simulink model "PMT_AI_Env_Version1_MatlabRL"  (R2025a)
settings: Solver=ode4  StartTime=0.0  StopTime=10  FixedStep=0.00001  RelTol=1e-3
libraries: instrumentlib x2, slpidlib x1
settings Model: Creator=30623  LastModifiedBy=Administrator

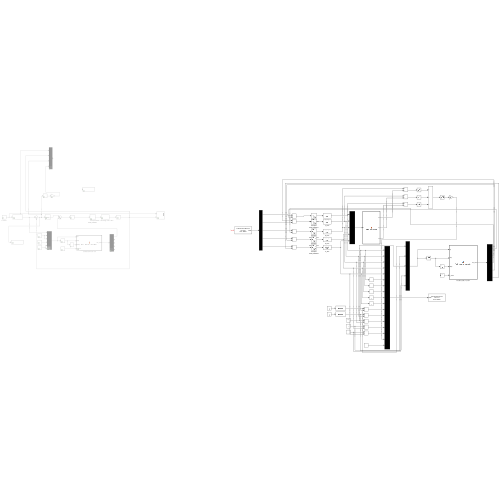
[thumbnail: Simulink's stored preview of the top-level diagram]
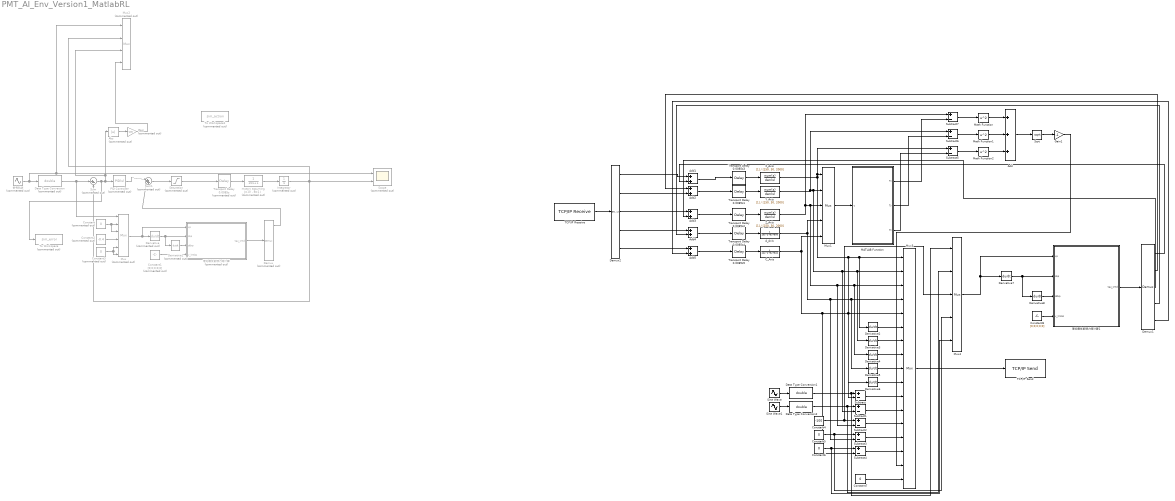
== system PMT_AI_Env_Version1_MatlabRL ==
  A_Axis : TransferFcn  Denominator=[20, 5, 500]
  Abs : Abs  Commented=on  SaturateOnIntegerOverflow=off
  Add : Sum  Inputs=+++
  Add{1..5} (5 alike) : Sum
  C_Axis : TransferFcn  Denominator=[20, 5, 500]
  Constant : Constant  Commented=on  Value=0
  Constant1 : Constant  Commented=on  Value=[0;0;0;0;0]
  Constant2 : Constant  Commented=on  Value=-0.4
  Constant3 : Constant  Commented=on  Value=0
  Constant4 : Constant  Value=-100
  Constant5 : Constant  Value=0
  Constant6 : Constant  Value=0
  Constant7 : Constant  Value=0
  Constant8 : Constant  Value=[0;0;0;0;0]
  Data Type Conversion : DataTypeConversion  Commented=on  OutDataTypeStr=double  SaturateOnIntegerOverflow=off  RndMeth=Floor
  Data Type Conversion1 : DataTypeConversion  OutDataTypeStr=double  SaturateOnIntegerOverflow=off  RndMeth=Floor
  Data Type Conversion2 : DataTypeConversion  OutDataTypeStr=double  SaturateOnIntegerOverflow=off  RndMeth=Floor
  Demux : Demux  Commented=on  Outputs=5
  Demux1 : Demux  Outputs=5
  Demux2 : Demux  Outputs=5
  Derivative : Derivative  Commented=on
  Derivative1 : Derivative  Commented=on
  Derivative{2..8} (7 alike) : Derivative
  Gain : Gain  Commented=on  Gain=-100
  Gain1 : Gain  Gain=-1
  Integrator : Integrator  Commented=on
  MATLAB Function : MATLAB Function  TreatAsAtomicUnit=on
  Math Function : Math  Operator=square
  Math Function1 : Math  Operator=square
  Math Function2 : Math  Operator=square
  Mux : Mux  Commented=on  Inputs=6
  Mux1 : Mux  Inputs=5
  Mux2 : Mux  Commented=on
  Mux3 : Mux  Inputs=17
  Mux4 : Mux  Inputs=5
  PID Controller : slpidlib/PID Controller  Commented=on  Controller=PID  Form=Parallel  TimeDomain=Continuous-time  UseExternalTs=off  SampleTime=-1  IntegratorMethod=Forward Euler  FilterMethod=Forward Euler  ControllerParametersSource=internal  P=1  I=1  UseKiTs=off  D=0  UseExternalDerivativeSource=off  N=100  UseFilter=on  TunerSelectOption=Transfer Function Based (PID Tuner App)  InitialConditionSource=internal  InitialConditionForIntegrator=0  InitialConditionForFilter=0  DifferentiatorICPrevScaledInput=0  ExternalReset=none  TrackingMode=off  Kt=1  LimitOutput=off  SatLimitsSource=internal  UpperSaturationLimit=inf  LowerSaturationLimit=-inf  LinearizeAsGain=on  AntiWindupMode=none  Kb=1  LimitIntegrator=off  UpperIntegratorSaturationLimit=inf  LowerIntegratorSaturationLimit=-inf  POutMin=[]  POutMax=[]  IOutMin=[]  IOutMax=[]  DOutMin=[]  DOutMax=[]  NOutMin=[]  NOutMax=[]  SumOutMin=[]  SumOutMax=[]  SaturationOutMin=[]  SaturationOutMax=[]  PParamMin=[]  PParamMax=[]  IParamMin=[]  IParamMax=[]  DParamMin=[]  DParamMax=[]  NParamMin=[]  NParamMax=[]  KbParamMin=[]  KbParamMax=[]  KtParamMin=[]  KtParamMax=[]  KbOutMin=[]  KbOutMax=[]  KtOutMin=[]  KtOutMax=[]  IntegratorOutMin=[]  IntegratorOutMax=[]  FilterOutMin=[]  FilterOutMax=[]  SumI1OutMin=[]  SumI1OutMax=[]  SumI2OutMin=[]  SumI2OutMax=[]  SumI3OutMin=[]  SumI3OutMax=[]  SumI4OutMin=[]  SumI4OutMax=[]  SumDOutMin=[]  SumDOutMax=[]  DifferentiatorOutMin=[]  DifferentiatorOutMax=[]  FilterDiffOutCoefMin=[]  FilterDiffOutCoefMax=[]  ReciprocalOutMin=[]  ReciprocalOutMax=[]  SumDenOutMin=[]  SumDenOutMax=[]  SumNumOutMin=[]  SumNumOutMax=[]  DivideOutMin=[]  DivideOutMax=[]  UdiffTsProdOutMin=[]  UdiffTsProdOutMax=[]  NTsProdOutMin=[]  NTsProdOutMax=[]  UintegralTsProdOutMin=[]  UintegralTsProdOutMax=[]  UngainTsProdOutMin=[]  UngainTsProdOutMax=[]  ClampingZeroOutDataTypeStr=Inherit: Inherit via back propagation  ClampingZeroOutMin=[]  ClampingZeroOutMax=[]  FilterDenConstantOutDataTypeStr=Inherit: Inherit via back propagation  FilterDenConstantOutMin=[]  FilterDenConstantOutMax=[]  PCopyOutDataTypeStr=Inherit: Inherit via back propagation  PCopyOutMin=[]  PCopyOutMax=[]  NCopyOutDataTypeStr=Inherit: Inherit via back propagation  NCopyOutMin=[]  NCopyOutMax=[]  IntegratorContinuousStateAttributes=''  IntegratorStateMustResolveToSignalObject=off  IntegratorRTWStateStorageClass=Auto  FilterContinuousStateAttributes=''  FilterStateMustResolveToSignalObject=off  FilterRTWStateStorageClass=Auto  ParallelPVariant=InternalParameters  IdealPVariant=Disabled  IVariant=InternalParameters  DVariant=InternalParameters  IntegratorVariant=Continuous  SatVariant=Disabled  AWVariant=Passthrough  PCopyVariant=Disabled  TRVariant=Disabled  FdbkBlocksVariant=Forward  IdealPFdbkVariant=Disabled  SatFdbkVariant=Disabled  DerivativeFilterVariant=ContFilter  NVariant=InternalParameters  NCopyVariant=Disabled  FilterICVariant=InternalICsFilter  IntegratorICVariant=InternalICs  ExternalResetVariant=Disabled  TRSumVariant=Passthrough  SumFdbkVariant=Disabled  SumVariant=Sum_PID  TsampFilterVariant=InternalTs  TsampNgainVariant=Passthrough  TsampIntegralVariant=Disabled_SignalSpec  ExternalSaturationOutDataTypeStr=Inherit: Same as second input  DerivativeSourceVariant=ErrorSignal  PreIntVariant=InternalPreInt
  Saturation : Saturate  Commented=on  UpperLimit=500  LowerLimit=-500
  Scope : Scope  Commented=on  NumInputPorts=2
      settings: ActiveDisplayYMinimum=-50413.733349400849  ActiveDisplayYMaximum=34151.372945794108
  Sine Wave : Sin  SampleTime=0
  Sine Wave1 : Sin  SampleTime=0
  Sqrt : Sqrt
  Subtract{,1..7} (8 alike) : Sum  Inputs=+-
  Sum : Sum  Commented=on  Inputs=|+-
  Sum1 : Sum  Commented=on  Inputs=|+++
  TCP/IP Receive : instrumentlib/TCP//IP Receive  Host=127.0.0.1  Port=50001  DataSize=5  DataType=double  ASCIIFormatting=%f  Terminator=LF  CustomTerminator=10  ByteOrder=big-endian  EnableBlockingMode=on  Timeout=30  SampleTime=0.01  SimulateUsing=Interpreted execution
  TCP/IP Send : instrumentlib/TCP//IP Send  Host=127.0.0.1  Port=50000  ByteOrder=big-endian  EnableBlockingMode=on  Timeout=10  TransferDelay=on  SimulateUsing=Interpreted execution
  To Workspace : ToWorkspace  Commented=on  VariableName=sim_error  SaveFormat=Timeseries  SampleTime=-1
  To Workspace1 : ToWorkspace  Commented=on  VariableName=sim_action  SaveFormat=Timeseries  SampleTime=-1
  Transport Delay 0.0085s : TransportDelay  Commented=on  DelayTime=0.00875
  Transport Delay 0.0085s{1..5} (5 alike) : TransportDelay  DelayTime=0.00875
  X_Axis : TransferFcn  Denominator=[150, 30, 2000]
  Y_Axis : TransferFcn  Denominator=[150, 30, 2000]
  Z_Axis : TransferFcn  Denominator=[150, 30, 2000]
  motor（assuming J=10，B=1） : TransferFcn  Commented=on  Denominator=[10 1]
  参考轨迹 : Sin  Commented=on  Amplitude=0.05  Frequency=2  SampleTime=0
  理论最优前馈力矩计算 : MATLAB Function  Commented=on  TreatAsAtomicUnit=on
  理论最优前馈力矩计算1 : MATLAB Function  TreatAsAtomicUnit=on
  wires:
  Transport Delay 0.0085s/1 -> motor（assuming J=10，B=1）/1
  Data Type Conversion/1 -> Mux/1, Sum/1
  Sum/1 -> To Workspace/1, Abs/1, Mux2/3, PID Controller/1
  motor（assuming J=10，B=1）/1 -> Integrator/1
  Integrator/1 -> Mux2/2, Sum/2, Scope/2
  PID Controller/1 -> Sum1/1
  Constant/1 -> Mux/3, Mux/2
  Mux/1 -> 理论最优前馈力矩计算/1(xp), Derivative/1
  Derivative/1 -> Derivative1/1, 理论最优前馈力矩计算/2(dxp)
  Derivative1/1 -> 理论最优前馈力矩计算/3(ddxp)
  Constant1/1 -> 理论最优前馈力矩计算/4(v_limbs)
  理论最优前馈力矩计算/1(tau_cmd) -> Demux/1
  Demux/1 -> Sum1/2
  参考轨迹/1 -> Mux2/1, Scope/1, Data Type Conversion/1
  Constant2/1 -> Mux/4
  Constant3/1 -> Mux/6, Mux/5
  Sum1/1 -> Saturation/1
  Saturation/1 -> Transport Delay 0.0085s/1
  Abs/1 -> Gain/1
  Gain/1 -> Mux2/4
  Z_Axis/1 -> Subtract7/1, Subtract2/2, Derivative4/1, Mux3/3, Mux1/3
  A_Axis/1 -> Mux1/4, Subtract3/2, Derivative5/1, Mux3/4
  C_Axis/1 -> Mux1/5, Subtract4/2, Derivative6/1, Mux3/5
  Mux1/1 -> MATLAB Function/1(u)
  X_Axis/1 -> Subtract5/1, Mux1/1, Subtract/2, Derivative2/1, Mux3/1
  Y_Axis/1 -> Mux1/2, Subtract1/2, Derivative3/1, Mux3/2, Subtract6/1
  Transport Delay 0.0085s3/1 -> X_Axis/1
  Transport Delay 0.0085s1/1 -> Y_Axis/1
  Transport Delay 0.0085s2/1 -> Z_Axis/1
  Transport Delay 0.0085s4/1 -> A_Axis/1
  Transport Delay 0.0085s5/1 -> C_Axis/1
  Derivative2/1 -> Mux3/6
  Derivative3/1 -> Mux3/7
  Derivative4/1 -> Mux3/8
  Derivative5/1 -> Mux3/9
  Derivative6/1 -> Mux3/10
  Sine Wave/1 -> Data Type Conversion1/1
  Constant4/1 -> Mux4/3, Subtract2/1
  Constant5/1 -> Mux4/4, Subtract3/1
  Constant6/1 -> Mux4/5, Subtract4/1
  Subtract/1 -> Mux3/11
  Subtract1/1 -> Mux3/12
  Subtract2/1 -> Mux3/13
  Subtract3/1 -> Mux3/14
  Subtract4/1 -> Mux3/15
  MATLAB Function/1(Tx) -> Subtract7/2
  MATLAB Function/2(Ty) -> Subtract6/2
  MATLAB Function/3(Tz) -> Subtract5/2
  Subtract7/1 -> Math Function/1
  Subtract6/1 -> Math Function1/1
  Subtract5/1 -> Math Function2/1
  Math Function/1 -> Add/1
  Math Function1/1 -> Add/2
  Math Function2/1 -> Add/3
  Add/1 -> Sqrt/1
  Sqrt/1 -> Gain1/1
  Gain1/1 -> Mux3/16
  Constant7/1 -> Mux3/17
  Mux3/1 -> TCP/IP Send/1
  Mux4/1 -> 理论最优前馈力矩计算1/1(xp), Derivative7/1
  Derivative7/1 -> Derivative8/1, 理论最优前馈力矩计算1/2(dxp)
  Derivative8/1 -> 理论最优前馈力矩计算1/3(ddxp)
  Constant8/1 -> 理论最优前馈力矩计算1/4(v_limbs)
  理论最优前馈力矩计算1/1(tau_cmd) -> Demux1/1
  Demux1/1 -> Add1/2
  Add1/1 -> Transport Delay 0.0085s3/1
  Demux1/2 -> Add2/1
  Add2/1 -> Transport Delay 0.0085s1/1
  Add3/1 -> Transport Delay 0.0085s2/1
  Add4/1 -> Transport Delay 0.0085s4/1
  Add5/1 -> Transport Delay 0.0085s5/1
  Demux1/3 -> Add3/2
  Demux1/4 -> Add4/2
  Demux1/5 -> Add5/2
  Data Type Conversion1/1 -> Mux4/1, Subtract/1
  Data Type Conversion2/1 -> Mux4/2, Subtract1/1
  Sine Wave1/1 -> Data Type Conversion2/1
  ? -> ?
  TCP/IP Receive/1 -> Demux2/1
  Demux2/1 -> Add1/1
  Demux2/2 -> Add2/2
  Demux2/3 -> Add3/1
  Demux2/4 -> Add4/1
  Demux2/5 -> Add5/1

== matlab function PMT_AI_Env_Version1_MatlabRL/MATLAB Function ==
  data: u input; Tx output; Ty output; Tz output
function [Tx, Ty, Tz] = FiveAxisKinematics(u)
    % 解析输入的 5 个实际物理量
    x = u(1); y = u(2); z = u(3); 
    a = u(4); c = u(5);
    
    % --- D-H 齐次变换矩阵推导 (基于 AC 摇篮台机床) ---
    % 1. 直线平移矩阵
    Trans = [1 0 0 x;
             0 1 0 y;
             0 0 1 z;
             0 0 0 1];
             
    % 2. A 轴旋转矩阵 (绕 X 轴)
    RotA = [1       0        0 0;
            0  cos(a)  -sin(a) 0;
            0  sin(a)   cos(a) 0;
            0       0        0 1];
           
    % 3. C 轴旋转矩阵 (绕 Z 轴)
    RotC = [cos(c) -sin(c) 0 0;
            sin(c)  cos(c) 0 0;
            0       0      1 0;
            0       0      0 1];
           
    % 4. 运动链合成
    T_total = Trans * RotA * RotC; 
    
    % 5. 计算真实的刀尖点 (假设初始刀具长度为100mm，沿Z轴负方向)
    P_tool = T_total * [0; 0; -100; 1];
    
    % 输出三维空间中真实的刀尖点坐标
    Tx = P_tool(1);
    Ty = P_tool(2);
    Tz = P_tool(3);
end

== matlab function PMT_AI_Env_Version1_MatlabRL/理论最优前馈力矩计算 ==
  data: xp input; tau_cmd output; dxp input; ddxp input; v_limbs input
%理论最优前馈力矩计算
function tau_cmd = PMT_Dynamics_Controller(xp, dxp, ddxp, v_limbs)
    % 输入: 
    % xp: [x, y, z, phi, theta]' 动平台位姿 (T&T angles)
    % dxp: [v_x, v_y, v_z, w_x, w_y, w_z]' 动平台速度 
    % ddxp: [a_x, a_y, a_z, dw_x, dw_y, dw_z]' 动平台加速度 
    % v_limbs: [v1, v2, v3, v4, v5]' 五个驱动支链的实际线速度 (用于计算摩擦力) 
    % 输出:
    % tau_cmd: [tau1, tau2, tau3, tau4, tau5]' 五个伺服电机的目标前馈力矩
    % 定义反对称矩阵算子 S(v)，用于计算叉乘 
    S = @(v) [0, -v(3), v(2); v(3), 0, -v(1); -v(2), v(1), 0];
    
    %% 1. 物理与几何参数化
    % 动平台真实辨识惯性参数 (摘自解老师论文 Table 2) 
    m_p = 45.32; 
    mp_es = 8.384; 
    I_xx = 6.24e-4; I_yy = 6.24e-4; I_zz = 1.03e-4;
    I_p_matrix = diag([I_xx, I_yy, I_zz]); % 忽略极小的耦合项 
    g_vec = [0; 0; -9.81]; 
    
    % 驱动支链真实辨识摩擦力参数 (摘自论文 Table 1: [Tc, Ts, vs, Bv]) 
    Fric_Params = [
        186.21, 291.52, -1.87, 3.027; % Limb 1
        244.34, 372.97,  1.26, 3.766; % Limb 2
        187.89, 273.38,  1.35, 3.006; % Limb 3
        226.99, 314.07,  1.30, 3.489; % Limb 4
        224.82, 312.41,  2.69, 2.696  % Limb 5
    ];
    
    % 虚拟几何参数 (因原论文未公开，用于 DRL 环境预研构建)
    R_b = 0.5; % 基座分布半径 0.5m
    b = [
        0,  R_b*cos(pi/4), R_b*cos(3*pi/4), R_b*cos(5*pi/4), R_b*cos(7*pi/4);
        0,  R_b*sin(pi/4), R_b*sin(3*pi/4), R_b*sin(5*pi/4), R_b*sin(7*pi/4);
        0,  0,             0,               0,               0
    ];
    
    R_p = 0.15; % 动平台铰链分布半径 0.15m
    H_tool = -0.1; % 刀尖到平台铰链面的 Z 向距离
    p_local = [
        0,       R_p*cos(pi/4), R_p*cos(3*pi/4), R_p*cos(5*pi/4), R_p*cos(7*pi/4);
        0,       R_p*sin(pi/4), R_p*sin(3*pi/4), R_p*sin(5*pi/4), R_p*sin(7*pi/4);
        H_tool,  H_tool,        H_tool,          H_tool,          H_tool
    ];
    
    %% 2. 运动学正解与雅可比矩阵构建 
    % (1) 计算旋转矩阵 R (基于 T&T angles, Eq. A-1) 
    phi = xp(4); theta = xp(5);
    p_vec = [cos(phi)*sin(theta); sin(phi)*sin(theta); cos(theta)];
    
    % 依据原论文的投影法生成正交旋转矩阵 R 
    O_B1 = b(:,1); 
    n_vec = cross(O_B1, p_vec); 
    if norm(n_vec) < 1e-6
        n_vec = [1;0;0]; % 奇异保护
    else
        n_vec = n_vec / norm(n_vec);
    end
    o_vec = cross(p_vec, n_vec);
    R = [n_vec, o_vec, p_vec];
    
    % (2) 运动传递雅可比 J_t (5x6 矩阵) 
    J_t = zeros(5, 6); 
    l_unit_all = zeros(3, 5); % 保存单位方向向量备用
    L_all = zeros(1, 5);      % 保存支链长度备用
    p_global_all = zeros(3, 5); % 保存全局坐标备用
    for i = 1:5
        p_i_global = R * p_local(:, i); % Eq. A-2 
        p_global_all(:, i) = p_i_global;
        
        l_vec = (xp(1:3) + p_i_global) - b(:, i); % Eq. A-3 
        L_i = norm(l_vec);
        L_all(i) = L_i;
        l_unit = l_vec / L_i; % Eq. A-3 
        l_unit_all(:, i) = l_unit;
        
        J_t(i, :) = [l_unit', (cross(p_i_global, l_unit))']; % 组装 J_t 
    end
    
    % (3) 约束雅可比 J_c (1x6 矩阵，第一条 SPR 支链提供的一维约束) 
    J_c = [n_vec', (L_all(1) * cross(n_vec, l_unit_all(:,1)) + cross(p_global_all(:,1), n_vec))'];
    % 组装完整满秩雅可比矩阵 J_a (6x6 矩阵) 
    J_a = [J_t; J_c]; 
    
    %% 3. 动力学受力分析 (附录 A.2 解老师用到了虚功原理) 
    % (1) 动平台惯性力和重力 F_p (Eq. A-12) 
    w_p = dxp(4:6);   % 角速度
    dw_p = ddxp(4:6); % 角加速度
    a_c = ddxp(1:3);  % 线加速度
    
    F_p_trans = m_p * g_vec - m_p * a_c; 
    F_p_rot = -I_p_matrix * dw_p - cross(w_p, I_p_matrix * w_p);
    F_p = [F_p_trans; F_p_rot]; % 6x1 向量
    
    % (2) 支链惯性力简化 (为提高仿真速度，此处将支链质量等效附加到平台上)
    F_limbs_total = zeros(6, 1); 
    
    %% 4. 虚功反解理论刚体力矩 
    % 求解: J_a' * [tau_ideal; F_constraint] = - F_p 
   Tau_and_Constraint = pinv(J_a') * (-F_p - F_limbs_total);
    tau_ideal = Tau_and_Constraint(1:5); % 提取前5个主动电机的理论力矩
    
    %% 5. Stribeck 非线性摩擦力补偿 (Eq. 4) 
    f_friction = zeros(5, 1);
    for i = 1:5
        v = v_limbs(i);
        Tc = Fric_Params(i, 1);
        Ts = Fric_Params(i, 2);
        vs = Fric_Params(i, 3);
        Bv = Fric_Params(i, 4);
       
        f_friction(i) = (Tc + (Ts - Tc) * exp(-(v/vs)^2)) * sign(v) + Bv * v; 
    end
    
    %% 6. 输出最终前馈力矩指令 
    tau_cmd = tau_ideal + f_friction;
end

== matlab function PMT_AI_Env_Version1_MatlabRL/理论最优前馈力矩计算1 ==
  data: xp input; tau_cmd output; dxp input; ddxp input; v_limbs input
%理论最优前馈力矩计算
function tau_cmd = PMT_Dynamics_Controller(xp, dxp, ddxp, v_limbs)
    % 输入: 
    % xp: [x, y, z, phi, theta]' 动平台位姿 (T&T angles)
    % dxp: [v_x, v_y, v_z, dphi, dtheta]' 或 [v_x, v_y, v_z, w_x, w_y, w_z]' 动平台速度 
    % ddxp: [a_x, a_y, a_z, ddphi, ddtheta]' 或 [a_x, a_y, a_z, dw_x, dw_y, dw_z]' 动平台加速度 
    % v_limbs: [v1, v2, v3, v4, v5]' 五个驱动支链的实际线速度 (用于计算摩擦力) 
    % 输出:
    % tau_cmd: [tau1, tau2, tau3, tau4, tau5]' 五个伺服电机的目标前馈力矩
    
    % 定义反对称矩阵算子 S(v)，用于计算叉乘 
    S = @(v) [0, -v(3), v(2); v(3), 0, -v(1); -v(2), v(1), 0];
    
    %% 1. 物理与几何参数化
    % 动平台真实辨识惯性参数 (摘自解老师论文 Table 2) 
    m_p = 45.32; 
    mp_es = 8.384; 
    I_xx = 6.24e-4; I_yy = 6.24e-4; I_zz = 1.03e-4;
    I_p_matrix = diag([I_xx, I_yy, I_zz]); % 忽略极小的耦合项 
    g_vec = [0; 0; -9.81]; 
    
    % 驱动支链真实辨识摩擦力参数 (摘自论文 Table 1: [Tc, Ts, vs, Bv]) 
    Fric_Params = [
        186.21, 291.52, -1.87, 3.027; % Limb 1
        244.34, 372.97,  1.26, 3.766; % Limb 2
        187.89, 273.38,  1.35, 3.006; % Limb 3
        226.99, 314.07,  1.30, 3.489; % Limb 4
        224.82, 312.41,  2.69, 2.696  % Limb 5
    ];
    
    % 虚拟几何参数 (因原论文未公开，用于 DRL 环境预研构建)
    R_b = 0.5; % 基座分布半径 0.5m
    b = [
        0,  R_b*cos(pi/4), R_b*cos(3*pi/4), R_b*cos(5*pi/4), R_b*cos(7*pi/4);
        0,  R_b*sin(pi/4), R_b*sin(3*pi/4), R_b*sin(5*pi/4), R_b*sin(7*pi/4);
        0,  0,             0,               0,               0
    ];
    
    R_p = 0.15; % 动平台铰链分布半径 0.15m
    H_tool = -0.1; % 刀尖到平台铰链面的 Z 向距离
    p_local = [
        0,       R_p*cos(pi/4), R_p*cos(3*pi/4), R_p*cos(5*pi/4), R_p*cos(7*pi/4);
        0,       R_p*sin(pi/4), R_p*sin(3*pi/4), R_p*sin(5*pi/4), R_p*sin(7*pi/4);
        H_tool,  H_tool,        H_tool,          H_tool,          H_tool
    ];
    
    %% 2. 运动学正解与雅可比矩阵构建 
    % (1) 计算旋转矩阵 R (基于 T&T angles, Eq. A-1) 
    phi = xp(4); theta = xp(5);
    p_vec = [cos(phi)*sin(theta); sin(phi)*sin(theta); cos(theta)];
    
    % 依据原论文的投影法生成正交旋转矩阵 R 
    O_B1 = b(:,1); 
    n_vec = cross(O_B1, p_vec); 
    if norm(n_vec) < 1e-6
        n_vec = [1;0;0]; % 奇异保护
    else
        n_vec = n_vec / norm(n_vec);
    end
    o_vec = cross(p_vec, n_vec);
    R = [n_vec, o_vec, p_vec];
    
    % (2) 运动传递雅可比 J_t (5x6 矩阵) 
    J_t = zeros(5, 6); 
    l_unit_all = zeros(3, 5); % 保存单位方向向量备用
    L_all = zeros(1, 5);      % 保存支链长度备用
    p_global_all = zeros(3, 5); % 保存全局坐标备用
    for i = 1:5
        p_i_global = R * p_local(:, i); % Eq. A-2 
        p_global_all(:, i) = p_i_global;
        
        l_vec = (xp(1:3) + p_i_global) - b(:, i); % Eq. A-3 
        L_i = norm(l_vec);
        L_all(i) = L_i;
        l_unit = l_vec / L_i; % Eq. A-3 
        l_unit_all(:, i) = l_unit;
        
        J_t(i, :) = [l_unit', (cross(p_i_global, l_unit))']; % 组装 J_t 
    end
    
    % (3) 约束雅可比 J_c (1x6 矩阵，第一条 SPR 支链提供的一维约束) 
    J_c = [n_vec', (L_all(1) * cross(n_vec, l_unit_all(:,1)) + cross(p_global_all(:,1), n_vec))'];
    % 组装完整满秩雅可比矩阵 J_a (6x6 矩阵) 
    J_a = [J_t; J_c]; 
    
    %% 3. 动力学受力分析 
    % ----- 【修复区域：自适应维度转换】 -----
    % 判断速度输入维度
    if length(dxp) == 5
        % 如果输入是 5 维：[vx, vy, vz, dphi, dtheta]
        dphi = dxp(4); 
        dtheta = dxp(5);
        % 映射到 3D 空间角速度
        w_p = [0; 0; dphi] + dtheta * n_vec; 
    else
        % 如果输入已经是 6 维：[vx, vy, vz, wx, wy, wz]
        w_p = dxp(4:6);
    end

    % 判断加速度输入维度
    if length(ddxp) == 5
        a_c = ddxp(1:3);
        ddphi = ddxp(4);
        ddtheta = ddxp(5);
        % 映射到 3D 空间角加速度
        dw_p = [0; 0; ddphi] + ddtheta * n_vec; 
    else
        a_c = ddxp(1:3);
        dw_p = ddxp(4:6);
    end
    % -----------------------------------------

    F_p_trans = m_p * g_vec - m_p * a_c; 
    F_p_rot = -I_p_matrix * dw_p - cross(w_p, I_p_matrix * w_p);
    F_p = [F_p_trans; F_p_rot]; % 此时 F_p 稳定输出为 6x1 向量
    
    % (2) 支链惯性力简化 (为提高仿真速度，此处将支链质量等效附加到平台上)
    F_limbs_total = zeros(6, 1); 
    
    %% 4. 虚功反解理论刚体力矩 
    % 求解: J_a' * [tau_ideal; F_constraint] = - F_p 
    Tau_and_Constraint = pinv(J_a') * (-F_p - F_limbs_total);
    tau_ideal = Tau_and_Constraint(1:5); % 提取前5个主动电机的理论力矩
    
    %% 5. Stribeck 非线性摩擦力补偿 (Eq. 4) 
    f_friction = zeros(5, 1);
    for i = 1:5
        v = v_limbs(i);
        Tc = Fric_Params(i, 1);
        Ts = Fric_Params(i, 2);
        vs = Fric_Params(i, 3);
        Bv = Fric_Params(i, 4);
       
        f_friction(i) = (Tc + (Ts - Tc) * exp(-(v/vs)^2)) * sign(v) + Bv * v; 
    end
    
    %% 6. 输出最终前馈力矩指令 
    tau_cmd = tau_ideal + f_friction;
end
